simulink model "wzor_01"  (R2015a)
settings: Solver=ode5  SolverMode=SingleTasking  StartTime=0.0  StopTime=inf  FixedStep=0.01  RelTol=1e-3  AbsTol=1e-6
undefined symbols (not defined in the file or in its folder): GetBias, GetScaleCoeff
undefined symbols (not defined in the file): TankBaseAddress
settings Model: SimulationMode=external  CovSFcnEnable=off  ExtModeTrigDuration=150000  ExtModeTrigLevel=0.400000  Creator=jims  LastModifiedBy=Student
settings DataIOCC: ExternalInput=[]  InitialState=[]  LimitDataPoints=off  MaxDataPoints=5000  SignalLoggingSaveFormat=ModelDataLogs  SaveOutput=off  SaveTime=off  SignalLoggingName=sigsOut
settings OptimizationCC: BooleanDataType=off  ExpressionDepthLimit=2147483647  InitFltsAndDblsToZero=on
settings DebuggingCC: SaveWithParameterizedLinksMsg=none  UnderspecifiedInitializationDetection=Classic  MergeDetectMultiDrivingBlocksExec=none  SignalResolutionControl=TryResolveAllWithWarning  MultiTaskDSMMsg=warning  MultiTaskCondExecSysMsg=none  IntegerOverflowMsg=none  FcnCallInpInsideContextMsg=UseLocalSettings  StateNameClashWarn=warning  IntegerSaturationMsg=none
settings HardwareCC: ProdBitPerLong=64  ProdBitPerPointer=64  ProdIntDivRoundTo=Zero  ProdEndianess=LittleEndian  ProdWordSize=64  ProdHWDeviceType=Intel->x86-64  TargetBitPerLong=64  TargetBitPerPointer=64  TargetIntDivRoundTo=Zero  TargetEndianess=LittleEndian  TargetWordSize=64  TargetHWDeviceType=Intel->x86-64
settings RTWCC: SystemTargetFile=rtwin.tlc  TemplateMakefile=rtwin.tmf  Description=Real-Time Windows Target  RTWCompilerOptimization=on
settings CodeAppCC: MaxIdLength=95
settings RTWinTargetCC: TargetPreCompLibLocation=C:\Program Files\MATLAB\R2015aSP1\toolbox\sldrt\lib\win64

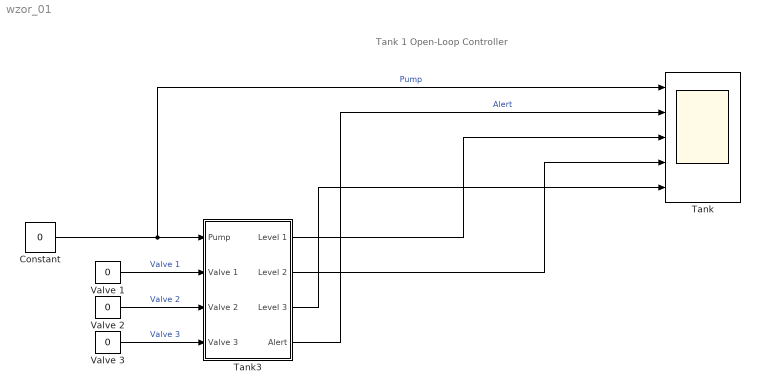
== system wzor_01 ==
  note: Tank 1 Open-Loop Controller
  Constant : Constant  Value=0
  Tank : Scope  NumInputPorts=5
      settings: TimeRange=12  YMin=-40~-1~1.5~1.3~0.5  YMax=30~1~3.25~2.5~2.25  SaveName=h_2  MaxDataPoints=150000  Decimation=10
  Tank3 : Subsystem  mask{BaseAddress=TankBaseAddress, T0=0.01}
      mask prompts: BaseAddress "Base Address:"; T0 "Sampling Period:"
      mask Display: image(imread('MultiTank.bmp'))
  Valve 1 : Constant  Value=0
  Valve 2 : Constant  Value=0
  Valve 3 : Constant  Value=0
  wires:
  Valve 3/1 -> Tank3/4(Valve 3)  "Valve 3"
  Valve 1/1 -> Tank3/2(Valve 1)  "Valve 1"
  Valve 2/1 -> Tank3/3(Valve 2)  "Valve 2"
  Tank3/4(Alert) -> Tank/2  "Alert"
  Tank3/2(Level 2) -> Tank/4
  Tank3/3(Level 3) -> Tank/5
  Tank3/1(Level 1) -> Tank/3
  Constant/1 -> Tank/1, Tank3/1(Pump)  "Pump"

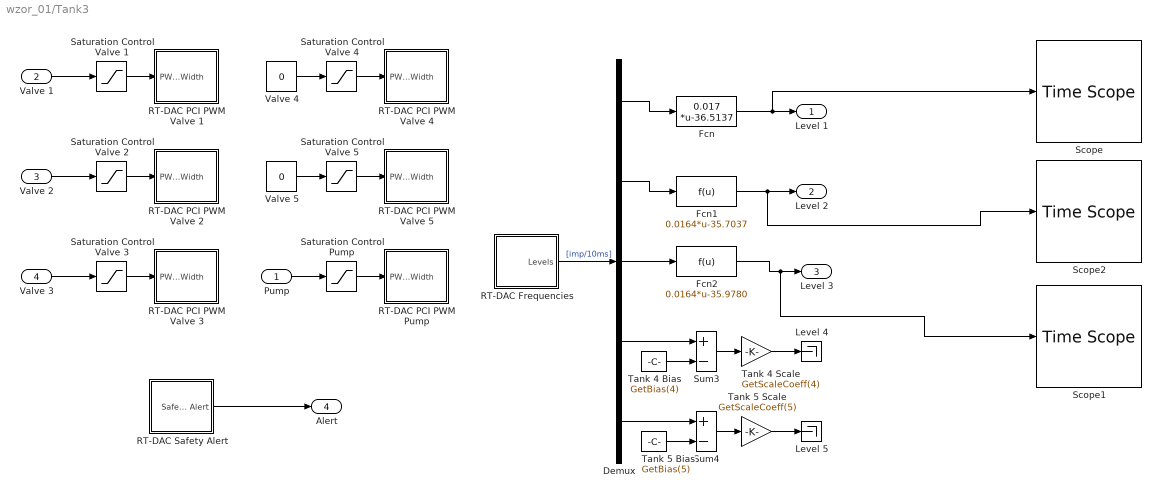
== system wzor_01/Tank3 ==
  Pump : Inport
  Valve 1 : Inport  Port=2
  Valve 2 : Inport  Port=3
  Valve 3 : Inport  Port=4
  Demux : Demux  Outputs=5
  Fcn : Fcn  Expr=0.017 *u-36.5137
  Fcn1 : Fcn  Expr=0.0164*u-35.7037
  Fcn2 : Fcn  Expr=0.0164*u-35.9780
  Level 4 : Terminator
  Level 5 : Terminator
  RT-DAC Frequencies : Subsystem  mask(Analog Input Module){BaseAddress=BaseAddress, T0=T0}
      mask prompts: BaseAddress "Base Address:"; T0 "Sample Time (sec):"
      mask help: RT-DAC PCI Device Driver
      mask Help: Set up each field for your specific hardware configuration.
      mask Display: plot(0,0,100,100,[90,80,80,11,11],[90,90,20,20,80],[11,80],[80,80],[80,80],[20,14],[80,85,85,80],[45,45,66,66],[45,45,74,74],[20,13,13,20],[15,27,27,15,15],[75,75,26,26,75],[33,48,48,33,33],[75,75,55,55,75],[55,55,71,71,55],[55,75,75,55,55],[33,41,41,33,33],[50,50,27,27,50],[48,56,56,48,48],[50,50,27,27,50],[62,70,70,62,62],[50,50,27,27,50])
  RT-DAC Safety Alert : Subsystem  mask(Analog Input Module){BaseAddress=BaseAddress, T0=T0}
      mask prompts: BaseAddress "Base Address:"; T0 "Sample Time (sec):"
      mask help: RT-DAC PCI Device Driver
      mask Help: Set up each field for your specific hardware configuration.
      mask Display: plot(0,0,100,100,[90,80,80,11,11],[90,90,20,20,80],[11,80],[80,80],[80,80],[20,14],[80,85,85,80],[45,45,66,66],[45,45,74,74],[20,13,13,20],[15,27,27,15,15],[75,75,26,26,75],[33,48,48,33,33],[75,75,55,55,75],[55,55,71,71,55],[55,75,75,55,55],[33,41,41,33,33],[50,50,27,27,50],[48,56,56,48,48],[50,50,27,27,50],[62,70,70,62,62],[50,50,27,27,50])
  RT-DAC PCI PWM Pump : Subsystem  mask(PWM Module){BaseAddress=BaseAddress, ChanIdx=0, ChanMode=12 Bit, ChanPresc=1, SetOutputsFlag=on, SetOutputsValue=0, T0=T0}
      mask prompts: BaseAddress "IO Base Address:"; ChanIdx "Channel:"; ChanMode "Channel Mode:"; ChanPresc "Channel Prescaler:"; SetOutputsFlag "Set Outputs At Termination"; SetOutputsValue "Termination Outputs:"; T0 "Sample Time (sec):"
      mask help: RT-DAC PCI Device Driver
      mask Help: Set up each field for your specific hardware configuration.
      mask TypeOptions ChanIdx: 0 | 1 | 2 | 3 | 4 | 5
      mask TypeOptions ChanMode: 8 Bit | 12 Bit
      mask Display: plot(0,0,100,100,[90,80,80,11,11],[90,90,20,20,80],[11,80],[80,80],[80,80],[20,14],[80,85,85,80],[45,45,66,66],[45,45,74,74],[20,13,13,20],[15,27,27,15,15],[75,75,26,26,75],[33,48,48,33,33],[75,75,55,55,75],[55,55,71,71,55],[55,75,75,55,55],[33,41,41,33,33],[50,50,27,27,50],[48,56,56,48,48],[50,50,27,27,50],[62,70,70,62,62],[50,50,27,27,50])
  RT-DAC PCI PWM Valve 1 : Subsystem  mask(PWM Module){BaseAddress=BaseAddress, ChanIdx=3, ChanMode=12 Bit, ChanPresc=31, SetOutputsFlag=on, SetOutputsValue=0, T0=T0}
      mask prompts: BaseAddress "IO Base Address:"; ChanIdx "Channel:"; ChanMode "Channel Mode:"; ChanPresc "Channel Prescaler:"; SetOutputsFlag "Set Outputs At Termination"; SetOutputsValue "Termination Outputs:"; T0 "Sample Time (sec):"
      mask help: RT-DAC PCI Device Driver
      mask Help: Set up each field for your specific hardware configuration.
      mask TypeOptions ChanIdx: 0 | 1 | 2 | 3 | 4 | 5
      mask TypeOptions ChanMode: 8 Bit | 12 Bit
      mask Display: plot(0,0,100,100,[90,80,80,11,11],[90,90,20,20,80],[11,80],[80,80],[80,80],[20,14],[80,85,85,80],[45,45,66,66],[45,45,74,74],[20,13,13,20],[15,27,27,15,15],[75,75,26,26,75],[33,48,48,33,33],[75,75,55,55,75],[55,55,71,71,55],[55,75,75,55,55],[33,41,41,33,33],[50,50,27,27,50],[48,56,56,48,48],[50,50,27,27,50],[62,70,70,62,62],[50,50,27,27,50])
  RT-DAC PCI PWM Valve 2 : Subsystem  mask(PWM Module){BaseAddress=BaseAddress, ChanIdx=2, ChanMode=12 Bit, ChanPresc=31, SetOutputsFlag=on, SetOutputsValue=0, T0=T0}
      mask prompts: BaseAddress "IO Base Address:"; ChanIdx "Channel:"; ChanMode "Channel Mode:"; ChanPresc "Channel Prescaler:"; SetOutputsFlag "Set Outputs At Termination"; SetOutputsValue "Termination Outputs:"; T0 "Sample Time (sec):"
      mask help: RT-DAC PCI Device Driver
      mask Help: Set up each field for your specific hardware configuration.
      mask TypeOptions ChanIdx: 0 | 1 | 2 | 3 | 4 | 5
      mask TypeOptions ChanMode: 8 Bit | 12 Bit
      mask Display: plot(0,0,100,100,[90,80,80,11,11],[90,90,20,20,80],[11,80],[80,80],[80,80],[20,14],[80,85,85,80],[45,45,66,66],[45,45,74,74],[20,13,13,20],[15,27,27,15,15],[75,75,26,26,75],[33,48,48,33,33],[75,75,55,55,75],[55,55,71,71,55],[55,75,75,55,55],[33,41,41,33,33],[50,50,27,27,50],[48,56,56,48,48],[50,50,27,27,50],[62,70,70,62,62],[50,50,27,27,50])
  RT-DAC PCI PWM Valve 3 : Subsystem  mask(PWM Module){BaseAddress=BaseAddress, ChanIdx=1, ChanMode=12 Bit, ChanPresc=31, SetOutputsFlag=on, SetOutputsValue=0, T0=T0}
      mask prompts: BaseAddress "IO Base Address:"; ChanIdx "Channel:"; ChanMode "Channel Mode:"; ChanPresc "Channel Prescaler:"; SetOutputsFlag "Set Outputs At Termination"; SetOutputsValue "Termination Outputs:"; T0 "Sample Time (sec):"
      mask help: RT-DAC PCI Device Driver
      mask Help: Set up each field for your specific hardware configuration.
      mask TypeOptions ChanIdx: 0 | 1 | 2 | 3 | 4 | 5
      mask TypeOptions ChanMode: 8 Bit | 12 Bit
      mask Display: plot(0,0,100,100,[90,80,80,11,11],[90,90,20,20,80],[11,80],[80,80],[80,80],[20,14],[80,85,85,80],[45,45,66,66],[45,45,74,74],[20,13,13,20],[15,27,27,15,15],[75,75,26,26,75],[33,48,48,33,33],[75,75,55,55,75],[55,55,71,71,55],[55,75,75,55,55],[33,41,41,33,33],[50,50,27,27,50],[48,56,56,48,48],[50,50,27,27,50],[62,70,70,62,62],[50,50,27,27,50])
  RT-DAC PCI PWM Valve 4 : Subsystem  mask(PWM Module){BaseAddress=BaseAddress, ChanIdx=5, ChanMode=12 Bit, ChanPresc=31, SetOutputsFlag=on, SetOutputsValue=0, T0=T0}
      mask prompts: BaseAddress "IO Base Address:"; ChanIdx "Channel:"; ChanMode "Channel Mode:"; ChanPresc "Channel Prescaler:"; SetOutputsFlag "Set Outputs At Termination"; SetOutputsValue "Termination Outputs:"; T0 "Sample Time (sec):"
      mask help: RT-DAC PCI Device Driver
      mask Help: Set up each field for your specific hardware configuration.
      mask TypeOptions ChanIdx: 0 | 1 | 2 | 3 | 4 | 5
      mask TypeOptions ChanMode: 8 Bit | 12 Bit
      mask Display: plot(0,0,100,100,[90,80,80,11,11],[90,90,20,20,80],[11,80],[80,80],[80,80],[20,14],[80,85,85,80],[45,45,66,66],[45,45,74,74],[20,13,13,20],[15,27,27,15,15],[75,75,26,26,75],[33,48,48,33,33],[75,75,55,55,75],[55,55,71,71,55],[55,75,75,55,55],[33,41,41,33,33],[50,50,27,27,50],[48,56,56,48,48],[50,50,27,27,50],[62,70,70,62,62],[50,50,27,27,50])
  RT-DAC PCI PWM Valve 5 : Subsystem  mask(PWM Module){BaseAddress=BaseAddress, ChanIdx=4, ChanMode=12 Bit, ChanPresc=31, SetOutputsFlag=on, SetOutputsValue=0, T0=T0}
      mask prompts: BaseAddress "IO Base Address:"; ChanIdx "Channel:"; ChanMode "Channel Mode:"; ChanPresc "Channel Prescaler:"; SetOutputsFlag "Set Outputs At Termination"; SetOutputsValue "Termination Outputs:"; T0 "Sample Time (sec):"
      mask help: RT-DAC PCI Device Driver
      mask Help: Set up each field for your specific hardware configuration.
      mask TypeOptions ChanIdx: 0 | 1 | 2 | 3 | 4 | 5
      mask TypeOptions ChanMode: 8 Bit | 12 Bit
      mask Display: plot(0,0,100,100,[90,80,80,11,11],[90,90,20,20,80],[11,80],[80,80],[80,80],[20,14],[80,85,85,80],[45,45,66,66],[45,45,74,74],[20,13,13,20],[15,27,27,15,15],[75,75,26,26,75],[33,48,48,33,33],[75,75,55,55,75],[55,55,71,71,55],[55,75,75,55,55],[33,41,41,33,33],[50,50,27,27,50],[48,56,56,48,48],[50,50,27,27,50],[62,70,70,62,62],[50,50,27,27,50])
  Saturation Control Pump : Saturate  UpperLimit=1  LowerLimit=0
  Saturation Control Valve {1..5} (5 alike) : Saturate  UpperLimit=1  LowerLimit=0
  Scope : TimeScope
  Scope1 : TimeScope
  Scope2 : TimeScope
  Sum3 : Sum  Inputs=+-  SaturateOnIntegerOverflow=on  InputSameDT=on  OutDataTypeStr=Inherit: Same as first input
  Sum4 : Sum  Inputs=+-  SaturateOnIntegerOverflow=on  InputSameDT=on  OutDataTypeStr=Inherit: Same as first input
  Tank 4 Bias : Constant  Value=GetBias(4)
  Tank 4 Scale : Gain  Gain=GetScaleCoeff(4)  SaturateOnIntegerOverflow=on  OutDataTypeStr=Inherit: Same as input  ParamDataTypeStr=Inherit: Same as input
  Tank 5 Bias : Constant  Value=GetBias(5)
  Tank 5 Scale : Gain  Gain=GetScaleCoeff(5)  SaturateOnIntegerOverflow=on  OutDataTypeStr=Inherit: Same as input  ParamDataTypeStr=Inherit: Same as input
  Valve 4 : Constant  Value=0
  Valve 5 : Constant  Value=0
  Level 1 : Outport
  Level 2 : Outport  Port=2
  Level 3 : Outport  Port=3
  Alert : Outport  Port=4
  wires:
  Tank 5 Scale/1 -> Level 5/1
  Tank 4 Scale/1 -> Level 4/1
  RT-DAC Safety Alert/1(Safety Alert) -> Alert/1
  Sum3/1 -> Tank 4 Scale/1
  Sum4/1 -> Tank 5 Scale/1
  Tank 5 Bias/1 -> Sum4/2
  Tank 4 Bias/1 -> Sum3/2
  Demux/5 -> Sum4/1
  Demux/4 -> Sum3/1
  RT-DAC Frequencies/1(Levels) -> Demux/1  "[imp/10ms]"
  Valve 5/1 -> Saturation Control Valve 5/1
  Valve 4/1 -> Saturation Control Valve 4/1
  Valve 3/1 -> Saturation Control Valve 3/1
  Valve 2/1 -> Saturation Control Valve 2/1
  Pump/1 -> Saturation Control Pump/1
  Saturation Control Pump/1 -> RT-DAC PCI PWM Pump/1(PWM Width)
  Saturation Control Valve 5/1 -> RT-DAC PCI PWM Valve 5/1(PWM Width)
  Saturation Control Valve 4/1 -> RT-DAC PCI PWM Valve 4/1(PWM Width)
  Saturation Control Valve 3/1 -> RT-DAC PCI PWM Valve 3/1(PWM Width)
  Saturation Control Valve 2/1 -> RT-DAC PCI PWM Valve 2/1(PWM Width)
  Saturation Control Valve 1/1 -> RT-DAC PCI PWM Valve 1/1(PWM Width)
  Valve 1/1 -> Saturation Control Valve 1/1
  Demux/1 -> Fcn/1
  Fcn/1 -> Scope/1, Level 1/1
  Fcn1/1 -> Scope2/1, Level 2/1
  Demux/2 -> Fcn1/1
  Demux/3 -> Fcn2/1
  Fcn2/1 -> Scope1/1, Level 3/1

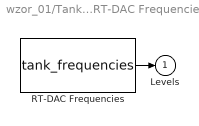
== system wzor_01/Tank3/RT-DAC Frequencies ==
  RT-DAC Frequencies : S-Function  FunctionName=tank_frequencies  Parameters=BaseAddress, T0
  Levels : Outport
  wires:
  RT-DAC Frequencies/1 -> Levels/1

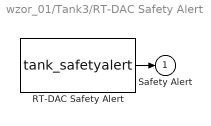
== system wzor_01/Tank3/RT-DAC Safety Alert ==
  RT-DAC Safety Alert : S-Function  FunctionName=tank_safetyalert  Parameters=BaseAddress, T0
  Safety Alert : Outport
  wires:
  RT-DAC Safety Alert/1 -> Safety Alert/1

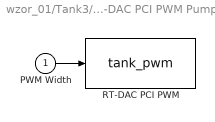
== system wzor_01/Tank3/RT-DAC PCI PWM Pump ==
  PWM Width : Inport
  "RT-DAC PCI PWM " : S-Function  FunctionName=tank_pwm  Parameters=BaseAddress, ChanIdx, ChanMode, ChanPresc, SetOutputsFlag, SetOutputsValue, T0
  wires:
  PWM Width/1 -> "RT-DAC PCI PWM "/1

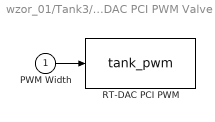
== system wzor_01/Tank3/RT-DAC PCI PWM Valve 1 ==
  PWM Width : Inport
  "RT-DAC PCI PWM " : S-Function  FunctionName=tank_pwm  Parameters=BaseAddress, ChanIdx, ChanMode, ChanPresc, SetOutputsFlag, SetOutputsValue, T0
  wires:
  PWM Width/1 -> "RT-DAC PCI PWM "/1

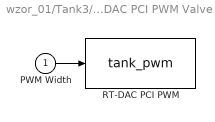
== system wzor_01/Tank3/RT-DAC PCI PWM Valve 2 ==
  PWM Width : Inport
  "RT-DAC PCI PWM " : S-Function  FunctionName=tank_pwm  Parameters=BaseAddress, ChanIdx, ChanMode, ChanPresc, SetOutputsFlag, SetOutputsValue, T0
  wires:
  PWM Width/1 -> "RT-DAC PCI PWM "/1

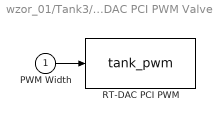
== system wzor_01/Tank3/RT-DAC PCI PWM Valve 3 ==
  PWM Width : Inport
  "RT-DAC PCI PWM " : S-Function  FunctionName=tank_pwm  Parameters=BaseAddress, ChanIdx, ChanMode, ChanPresc, SetOutputsFlag, SetOutputsValue, T0
  wires:
  PWM Width/1 -> "RT-DAC PCI PWM "/1

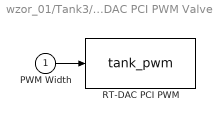
== system wzor_01/Tank3/RT-DAC PCI PWM Valve 4 ==
  PWM Width : Inport
  "RT-DAC PCI PWM " : S-Function  FunctionName=tank_pwm  Parameters=BaseAddress, ChanIdx, ChanMode, ChanPresc, SetOutputsFlag, SetOutputsValue, T0
  wires:
  PWM Width/1 -> "RT-DAC PCI PWM "/1

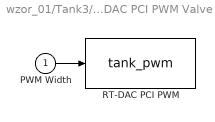
== system wzor_01/Tank3/RT-DAC PCI PWM Valve 5 ==
  PWM Width : Inport
  "RT-DAC PCI PWM " : S-Function  FunctionName=tank_pwm  Parameters=BaseAddress, ChanIdx, ChanMode, ChanPresc, SetOutputsFlag, SetOutputsValue, T0
  wires:
  PWM Width/1 -> "RT-DAC PCI PWM "/1
